simulink model "PI_check"  (R2018a)
settings: Solver=FixedStepAuto  StartTime=0.0  StopTime=10.0  FixedStep=0.01  RelTol=1e-3
libraries: simulink x1
settings Model: Creator=adiravishankara  LastModifiedBy=adiravishankara

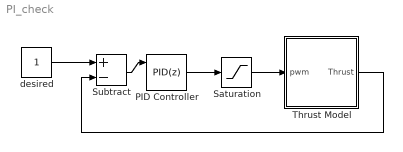
== system PI_check ==
  PID Controller : simulink/Continuous/PID Controller  Controller=PID  TimeDomain=Discrete-time  SampleTime=-1  IntegratorMethod=Forward Euler  FilterMethod=Forward Euler  Form=Parallel  UseFilter=on  ControllerParametersSource=internal  P=21.0398979422587  I=22.1641161959606  D=4.45675063345533  N=154.23857900008  InitialConditionSource=internal  InitialConditionForIntegrator=0  InitialConditionForFilter=0  ExternalReset=rising  LimitOutput=off  UpperSaturationLimit=inf  LowerSaturationLimit=-inf  LinearizeAsGain=on  AntiWindupMode=none  Kb=1  TrackingMode=off  Kt=1  PParamMin=[]  PParamMax=[]  IParamMin=[]  IParamMax=[]  DParamMin=[]  DParamMax=[]  NParamMin=[]  NParamMax=[]  KbParamMin=[]  KbParamMax=[]  KtParamMin=[]  KtParamMax=[]  POutMin=[]  POutMax=[]  IOutMin=[]  IOutMax=[]  DOutMin=[]  DOutMax=[]  NOutMin=[]  NOutMax=[]  KbOutMin=[]  KbOutMax=[]  KtOutMin=[]  KtOutMax=[]  IntegratorOutMin=[]  IntegratorOutMax=[]  FilterOutMin=[]  FilterOutMax=[]  SumOutMin=[]  SumOutMax=[]  SumI1OutMin=[]  SumI1OutMax=[]  SumI2OutMin=[]  SumI2OutMax=[]  SumI3OutMin=[]  SumI3OutMax=[]  SumDOutMin=[]  SumDOutMax=[]  SaturationOutMin=[]  SaturationOutMax=[]  IntegratorContinuousStateAttributes=''  IntegratorStateMustResolveToSignalObject=off  IntegratorRTWStateStorageClass=Auto  FilterContinuousStateAttributes=''  FilterStateMustResolveToSignalObject=off  FilterRTWStateStorageClass=Auto  DifferentiatorICPrevScaledInput=0  DifferentiatorOutMin=[]  DifferentiatorOutMax=[]  InitialConditionSetting=Output  FilterDiffOutCoefMin=[]  FilterDiffOutCoefMax=[]  SumDenOutMin=[]  SumDenOutMax=[]  SumNumOutMin=[]  SumNumOutMax=[]  ReciprocalOutMin=[]  ReciprocalOutMax=[]  DivideOutMin=[]  DivideOutMax=[]  TunerSelectOption=Transfer Function Based (PID Tuner App)
  Saturation : Saturate  UpperLimit=40  LowerLimit=0
  Subtract : Sum  Inputs=+-
  Thrust Model : Subsystem
  desired : Constant
  wires:
  PID Controller/1 -> Saturation/1
  Subtract/1 -> PID Controller/1
  Thrust Model/1(Thrust) -> Subtract/2
  Saturation/1 -> Thrust Model/1(pwm)
  desired/1 -> Subtract/1

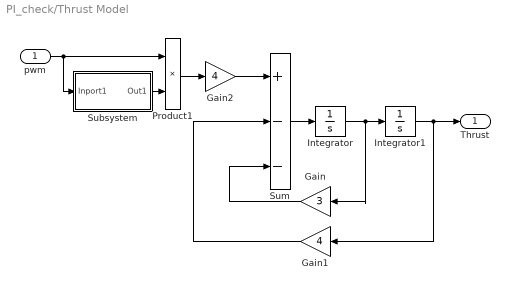
== system PI_check/Thrust Model ==
  pwm : Inport
  Gain : Gain  Gain=3
  Gain1 : Gain  Gain=4
  Gain2 : Gain  Gain=4
  Integrator : Integrator
  Integrator1 : Integrator
  Product1 : Product
  Subsystem : Subsystem
  Sum : Sum  Inputs=+--
  Thrust : Outport
  wires:
  Product1/1 -> Gain2/1
  pwm/1 -> Product1/1, Subsystem/1(Inport1)
  Integrator/1 -> Gain/1, Integrator1/1
  Subsystem/1(Out1) -> Product1/2
  Sum/1 -> Integrator/1
  Integrator1/1 -> Gain1/1, Thrust/1
  Gain/1 -> Sum/3
  Gain1/1 -> Sum/2
  Gain2/1 -> Sum/1

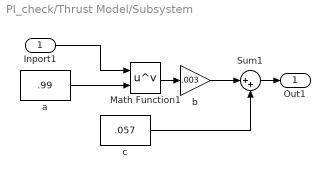
== system PI_check/Thrust Model/Subsystem ==
  Inport1 : Inport
  Math Function1 : Math  Operator=pow  SaturateOnIntegerOverflow=on
  Sum1 : Sum  Inputs=|++
  a : Constant  Value=.99
  b : Gain  Gain=.003
  c : Constant  Value=.057
  Out1 : Outport
  wires:
  a/1 -> Math Function1/2
  b/1 -> Sum1/1
  Inport1/1 -> Math Function1/1
  Math Function1/1 -> b/1
  Sum1/1 -> Out1/1
  c/1 -> Sum1/2
